simulink model "elevator"  (R2020a)
(part 3 of 38)

      mask DialogControl PLCBlockTitle Prompt: Examine If Closed (XIC)
  XIC3 : Subsystem  Priority=113  TreatAsAtomicUnit=on  mask{PLCOperandTag=F1PB, PLCBlockType=XIC, PLCPOUType=Contact, PLCOperandExpression=xxx_PLC_VAR_F1PB}
      mask prompts: PLCOperandTag "Operand Tag:"
      mask init:
      | slplc.callbacks.initInstruction(gcb);
      settings: AttributesFormatString=%<PLCOperandTag>
      mask Help: web([docroot '/plccoder/ref/xic' '.html']);
      mask DialogControl PLCBlockTitle Prompt: Examine If Closed (XIC)
  XIC30 : Subsystem  Priority=176  TreatAsAtomicUnit=on  mask{PLCOperandTag=F1PBHold, PLCBlockType=XIC, PLCPOUType=Contact, PLCOperandExpression=xxx_PLC_VAR_F1PBHold}
      mask prompts: PLCOperandTag "Operand Tag:"
      mask init:
      | slplc.callbacks.initInstruction(gcb);
      settings: AttributesFormatString=%<PLCOperandTag>
      mask Help: web([docroot '/plccoder/ref/xic' '.html']);
      mask DialogControl PLCBlockTitle Prompt: Examine If Closed (XIC)
  XIC31 : Subsystem  Priority=196  TreatAsAtomicUnit=on  mask{PLCOperandTag=StartHold, PLCBlockType=XIC, PLCPOUType=Contact, PLCOperandExpression=xxx_PLC_VAR_StartHold}
      mask prompts: PLCOperandTag "Operand Tag:"
      mask init:
      | slplc.callbacks.initInstruction(gcb);
      settings: AttributesFormatString=%<PLCOperandTag>
      mask Help: web([docroot '/plccoder/ref/xic' '.html']);
      mask DialogControl PLCBlockTitle Prompt: Examine If Closed (XIC)
  XIC32 : Subsystem  Priority=198  TreatAsAtomicUnit=on  mask{PLCOperandTag=LSTDIRUP, PLCBlockType=XIC, PLCPOUType=Contact, PLCOperandExpression=xxx_PLC_VAR_LSTDIRUP}
      mask prompts: PLCOperandTag "Operand Tag:"
      mask init:
      | slplc.callbacks.initInstruction(gcb);
      settings: AttributesFormatString=%<PLCOperandTag>
      mask Help: web([docroot '/plccoder/ref/xic' '.html']);
      mask DialogControl PLCBlockTitle Prompt: Examine If Closed (XIC)
  XIC33 : Subsystem  Priority=197  TreatAsAtomicUnit=on  mask{PLCOperandTag=GOINGUP, PLCBlockType=XIC, PLCPOUType=Contact, PLCOperandExpression=xxx_PLC_VAR_GOINGUP}
      mask prompts: PLCOperandTag "Operand Tag:"
      mask init:
      | slplc.callbacks.initInstruction(gcb);
      settings: AttributesFormatString=%<PLCOperandTag>
      mask Help: web([docroot '/plccoder/ref/xic' '.html']);
      mask DialogControl PLCBlockTitle Prompt: Examine If Closed (XIC)
  XIC34 : Subsystem  Priority=234  TreatAsAtomicUnit=on  mask{PLCOperandTag=MTRON, PLCBlockType=XIC, PLCPOUType=Contact, PLCOperandExpression=xxx_PLC_VAR_MTRON}
      mask prompts: PLCOperandTag "Operand Tag:"
      mask init:
      | slplc.callbacks.initInstruction(gcb);
      settings: AttributesFormatString=%<PLCOperandTag>
      mask Help: web([docroot '/plccoder/ref/xic' '.html']);
      mask DialogControl PLCBlockTitle Prompt: Examine If Closed (XIC)
  XIC35 : Subsystem  Priority=221  TreatAsAtomicUnit=on  mask{PLCOperandTag=F2PBHold, PLCBlockType=XIC, PLCPOUType=Contact, PLCOperandExpression=xxx_PLC_VAR_F2PBHold}
      mask prompts: PLCOperandTag "Operand Tag:"
      mask init:
      | slplc.callbacks.initInstruction(gcb);
      settings: AttributesFormatString=%<PLCOperandTag>
      mask Help: web([docroot '/plccoder/ref/xic' '.html']);
      mask DialogControl PLCBlockTitle Prompt: Examine If Closed (XIC)
  XIC36 : Subsystem  Priority=216  TreatAsAtomicUnit=on  mask{PLCOperandTag=F3DownBHold, PLCBlockType=XIC, PLCPOUType=Contact, PLCOperandExpression=xxx_PLC_VAR_F3DownBHold}
      mask prompts: PLCOperandTag "Operand Tag:"
      mask init:
      | slplc.callbacks.initInstruction(gcb);
      settings: AttributesFormatString=%<PLCOperandTag>
      mask Help: web([docroot '/plccoder/ref/xic' '.html']);
      mask DialogControl PLCBlockTitle Prompt: Examine If Closed (XIC)
  XIC37 : Subsystem  Priority=211  TreatAsAtomicUnit=on  mask{PLCOperandTag=F2PBHold, PLCBlockType=XIC, PLCPOUType=Contact, PLCOperandExpression=xxx_PLC_VAR_F2PBHold}
      mask prompts: PLCOperandTag "Operand Tag:"
      mask init:
      | slplc.callbacks.initInstruction(gcb);
      settings: AttributesFormatString=%<PLCOperandTag>
      mask Help: web([docroot '/plccoder/ref/xic' '.html']);
      mask DialogControl PLCBlockTitle Prompt: Examine If Closed (XIC)
  XIC38 : Subsystem  Priority=248  TreatAsAtomicUnit=on  mask{PLCOperandTag=MTRON, PLCBlockType=XIC, PLCPOUType=Contact, PLCOperandExpression=xxx_PLC_VAR_MTRON}
      mask prompts: PLCOperandTag "Operand Tag:"
      mask init:
      | slplc.callbacks.initInstruction(gcb);
      settings: AttributesFormatString=%<PLCOperandTag>
      mask Help: web([docroot '/plccoder/ref/xic' '.html']);
      mask DialogControl PLCBlockTitle Prompt: Examine If Closed (XIC)
  XIC39 : Subsystem  Priority=249  TreatAsAtomicUnit=on  mask{PLCOperandTag=RMPUPTRG, PLCBlockType=XIC, PLCPOUType=Contact, PLCOperandExpression=xxx_PLC_VAR_RMPUPTRG}
      mask prompts: PLCOperandTag "Operand Tag:"
      mask init:
      | slplc.callbacks.initInstruction(gcb);
      settings: AttributesFormatString=%<PLCOperandTag>
      mask Help: web([docroot '/plccoder/ref/xic' '.html']);
      mask DialogControl PLCBlockTitle Prompt: Examine If Closed (XIC)
  XIC4 : Subsystem  Priority=114  TreatAsAtomicUnit=on  mask{PLCOperandTag=F1PBHold, PLCBlockType=XIC, PLCPOUType=Contact, PLCOperandExpression=xxx_PLC_VAR_F1PBHold}
      mask prompts: PLCOperandTag "Operand Tag:"
      mask init:
      | slplc.callbacks.initInstruction(gcb);
      settings: AttributesFormatString=%<PLCOperandTag>
      mask Help: web([docroot '/plccoder/ref/xic' '.html']);
      mask DialogControl PLCBlockTitle Prompt: Examine If Closed (XIC)
  XIC40 : Subsystem  Priority=250  TreatAsAtomicUnit=on  mask{PLCOperandTag=RMPUP, PLCBlockType=XIC, PLCPOUType=Contact, PLCOperandExpression=xxx_PLC_VAR_RMPUP}
      mask prompts: PLCOperandTag "Operand Tag:"
      mask init:
      | slplc.callbacks.initInstruction(gcb);
      settings: AttributesFormatString=%<PLCOperandTag>
      mask Help: web([docroot '/plccoder/ref/xic' '.html']);
      mask DialogControl PLCBlockTitle Prompt: Examine If Closed (XIC)
  XIC41 : Subsystem  Priority=242  TreatAsAtomicUnit=on  mask{PLCOperandTag=SENCHK, PLCBlockType=XIC, PLCPOUType=Contact, PLCOperandExpression=xxx_PLC_VAR_SENCHK}
      mask prompts: PLCOperandTag "Operand Tag:"
      mask init:
      | slplc.callbacks.initInstruction(gcb);
      settings: AttributesFormatString=%<PLCOperandTag>
      mask Help: web([docroot '/plccoder/ref/xic' '.html']);
      mask DialogControl PLCBlockTitle Prompt: Examine If Closed (XIC)
  XIC42 : Subsystem  Priority=233  TreatAsAtomicUnit=on  mask{PLCOperandTag=StartHold, PLCBlockType=XIC, PLCPOUType=Contact, PLCOperandExpression=xxx_PLC_VAR_StartHold}
      mask prompts: PLCOperandTag "Operand Tag:"
      mask init:
      | slplc.callbacks.initInstruction(gcb);
      settings: AttributesFormatString=%<PLCOperandTag>
      mask Help: web([docroot '/plccoder/ref/xic' '.html']);
      mask DialogControl PLCBlockTitle Prompt: Examine If Closed (XIC)
  XIC43 : Subsystem  Priority=65  TreatAsAtomicUnit=on  mask{PLCOperandTag=TempS3LUp, PLCBlockType=XIC, PLCPOUType=Contact, PLCOperandExpression=xxx_PLC_VAR_TempS3LUp}
      mask prompts: PLCOperandTag "Operand Tag:"
      mask init:
      | slplc.callbacks.initInstruction(gcb);
      settings: AttributesFormatString=%<PLCOperandTag>
      mask Help: web([docroot '/plccoder/ref/xic' '.html']);
      mask DialogControl PLCBlockTitle Prompt: Examine If Closed (XIC)
  XIC44 : Subsystem  Priority=183  TreatAsAtomicUnit=on  mask{PLCOperandTag=MemoryGoUp, PLCBlockType=XIC, PLCPOUType=Contact, PLCOperandExpression=xxx_PLC_VAR_MemoryGoUp}
      mask prompts: PLCOperandTag "Operand Tag:"
      mask init:
      | slplc.callbacks.initInstruction(gcb);
      settings: AttributesFormatString=%<PLCOperandTag>
      mask Help: web([docroot '/plccoder/ref/xic' '.html']);
      mask DialogControl PLCBlockTitle Prompt: Examine If Closed (XIC)
  XIC45 : Subsystem  Priority=64  TreatAsAtomicUnit=on  mask{PLCOperandTag=StartHold, PLCBlockType=XIC, PLCPOUType=Contact, PLCOperandExpression=xxx_PLC_VAR_StartHold}
      mask prompts: PLCOperandTag "Operand Tag:"
      mask init:
      | slplc.callbacks.initInstruction(gcb);
      settings: AttributesFormatString=%<PLCOperandTag>
      mask Help: web([docroot '/plccoder/ref/xic' '.html']);
      mask DialogControl PLCBlockTitle Prompt: Examine If Closed (XIC)
  XIC46 : Subsystem  Priority=228  TreatAsAtomicUnit=on  mask{PLCOperandTag=S1H, PLCBlockType=XIC, PLCPOUType=Contact, PLCOperandExpression=xxx_PLC_VAR_S1H}
      mask prompts: PLCOperandTag "Operand Tag:"
      mask init:
      | slplc.callbacks.initInstruction(gcb);
      settings: AttributesFormatString=%<PLCOperandTag>
      mask Help: web([docroot '/plccoder/ref/xic' '.html']);
      mask DialogControl PLCBlockTitle Prompt: Examine If Closed (XIC)
  XIC47 : Subsystem  Priority=214  TreatAsAtomicUnit=on  mask{PLCOperandTag=S2L, PLCBlockType=XIC, PLCPOUType=Contact, PLCOperandExpression=xxx_PLC_VAR_S2L}
      mask prompts: PLCOperandTag "Operand Tag:"
      mask init:
      | slplc.callbacks.initInstruction(gcb);
      settings: AttributesFormatString=%<PLCOperandTag>
      mask Help: web([docroot '/plccoder/ref/xic' '.html']);
      mask DialogControl PLCBlockTitle Prompt: Examine If Closed (XIC)
  XIC48 : Subsystem  Priority=222  TreatAsAtomicUnit=on  mask{PLCOperandTag=F2UpDownBHold, PLCBlockType=XIC, PLCPOUType=Contact, PLCOperandExpression=xxx_PLC_VAR_F2UpDownBHold}
      mask prompts: PLCOperandTag "Operand Tag:"
      mask init:
      | slplc.callbacks.initInstruction(gcb);
      settings: AttributesFormatString=%<PLCOperandTag>
      mask Help: web([docroot '/plccoder/ref/xic' '.html']);
      mask DialogControl PLCBlockTitle Prompt: Examine If Closed (XIC)
  XIC49 : Subsystem  Priority=218  TreatAsAtomicUnit=on  mask{PLCOperandTag=S3L, PLCBlockType=XIC, PLCPOUType=Contact, PLCOperandExpression=xxx_PLC_VAR_S3L}
      mask prompts: PLCOperandTag "Operand Tag:"
      mask init:
      | slplc.callbacks.initInstruction(gcb);
      settings: AttributesFormatString=%<PLCOperandTag>
      mask Help: web([docroot '/plccoder/ref/xic' '.html']);
      mask DialogControl PLCBlockTitle Prompt: Examine If Closed (XIC)
  XIC5 : Subsystem  Priority=140  TreatAsAtomicUnit=on  mask{PLCOperandTag=StartHold, PLCBlockType=XIC, PLCPOUType=Contact, PLCOperandExpression=xxx_PLC_VAR_StartHold}
      mask prompts: PLCOperandTag "Operand Tag:"
      mask init:
      | slplc.callbacks.initInstruction(gcb);
      settings: AttributesFormatString=%<PLCOperandTag>
      mask Help: web([docroot '/plccoder/ref/xic' '.html']);
      mask DialogControl PLCBlockTitle Prompt: Examine If Closed (XIC)
  XIC50 : Subsystem  Priority=224  TreatAsAtomicUnit=on  mask{PLCOperandTag=S2H, PLCBlockType=XIC, PLCPOUType=Contact, PLCOperandExpression=xxx_PLC_VAR_S2H}
      mask prompts: PLCOperandTag "Operand Tag:"
      mask init:
      | slplc.callbacks.initInstruction(gcb);
      settings: AttributesFormatString=%<PLCOperandTag>
      mask Help: web([docroot '/plccoder/ref/xic' '.html']);
      mask DialogControl PLCBlockTitle Prompt: Examine If Closed (XIC)
  XIC51 : Subsystem  Priority=225  TreatAsAtomicUnit=on  mask{PLCOperandTag=F1PBHold, PLCBlockType=XIC, PLCPOUType=Contact, PLCOperandExpression=xxx_PLC_VAR_F1PBHold}
      mask prompts: PLCOperandTag "Operand Tag:"
      mask init:
      | slplc.callbacks.initInstruction(gcb);
      settings: AttributesFormatString=%<PLCOperandTag>
      mask Help: web([docroot '/plccoder/ref/xic' '.html']);
      mask DialogControl PLCBlockTitle Prompt: Examine If Closed (XIC)
  XIC52 : Subsystem  Priority=212  TreatAsAtomicUnit=on  mask{PLCOperandTag=F2UpDownBHold, PLCBlockType=XIC, PLCPOUType=Contact, PLCOperandExpression=xxx_PLC_VAR_F2UpDownBHold}
      mask prompts: PLCOperandTag "Operand Tag:"
      mask init:
      | slplc.callbacks.initInstruction(gcb);
      settings: AttributesFormatString=%<PLCOperandTag>
      mask Help: web([docroot '/plccoder/ref/xic' '.html']);
      mask DialogControl PLCBlockTitle Prompt: Examine If Closed (XIC)
  XIC53 : Subsystem  Priority=210  TreatAsAtomicUnit=on  mask{PLCOperandTag=GOINGUP, PLCBlockType=XIC, PLCPOUType=Contact, PLCOperandExpression=xxx_PLC_VAR_GOINGUP}
      mask prompts: PLCOperandTag "Operand Tag:"
      mask init:
      | slplc.callbacks.initInstruction(gcb);
      settings: AttributesFormatString=%<PLCOperandTag>
      mask Help: web([docroot '/plccoder/ref/xic' '.html']);
      mask DialogControl PLCBlockTitle Prompt: Examine If Closed (XIC)
  XIC54 : Subsystem  Priority=215  TreatAsAtomicUnit=on  mask{PLCOperandTag=F3PBHold, PLCBlockType=XIC, PLCPOUType=Contact, PLCOperandExpression=xxx_PLC_VAR_F3PBHold}
      mask prompts: PLCOperandTag "Operand Tag:"
      mask init:
      | slplc.callbacks.initInstruction(gcb);
      settings: AttributesFormatString=%<PLCOperandTag>
      mask Help: web([docroot '/plccoder/ref/xic' '.html']);
      mask DialogControl PLCBlockTitle Prompt: Examine If Closed (XIC)
  XIC55 : Subsystem  Priority=220  TreatAsAtomicUnit=on  mask{PLCOperandTag=GOINGDN, PLCBlockType=XIC, PLCPOUType=Contact, PLCOperandExpression=xxx_PLC_VAR_GOINGDN}
      mask prompts: PLCOperandTag "Operand Tag:"
      mask init:
      | slplc.callbacks.initInstruction(gcb);
      settings: AttributesFormatString=%<PLCOperandTag>
      mask Help: web([docroot '/plccoder/ref/xic' '.html']);
      mask DialogControl PLCBlockTitle Prompt: Examine If Closed (XIC)
  XIC56 : Subsystem  Priority=209  TreatAsAtomicUnit=on  mask{PLCOperandTag=StartHold, PLCBlockType=XIC, PLCPOUType=Contact, PLCOperandExpression=xxx_PLC_VAR_StartHold}
      mask prompts: PLCOperandTag "Operand Tag:"
      mask init:
      | slplc.callbacks.initInstruction(gcb);
      settings: AttributesFormatString=%<PLCOperandTag>
      mask Help: web([docroot '/plccoder/ref/xic' '.html']);
      mask DialogControl PLCBlockTitle Prompt: Examine If Closed (XIC)
  XIC57 : Subsystem  Priority=226  TreatAsAtomicUnit=on  mask{PLCOperandTag=F1UpBHold, PLCBlockType=XIC, PLCPOUType=Contact, PLCOperandExpression=xxx_PLC_VAR_F1UpBHold}
      mask prompts: PLCOperandTag "Operand Tag:"
      mask init:
      | slplc.callbacks.initInstruction(gcb);
      settings: AttributesFormatString=%<PLCOperandTag>
      mask Help: web([docroot '/plccoder/ref/xic' '.html']);
      mask DialogControl PLCBlockTitle Prompt: Examine If Closed (XIC)
  XIC58 : Subsystem  Priority=8  TreatAsAtomicUnit=on  mask{PLCOperandTag=StartHold, PLCBlockType=XIC, PLCPOUType=Contact, PLCOperandExpression=xxx_PLC_VAR_StartHold}
      mask prompts: PLCOperandTag "Operand Tag:"
      mask init:
      | slplc.callbacks.initInstruction(gcb);
      settings: AttributesFormatString=%<PLCOperandTag>
      mask Help: web([docroot '/plccoder/ref/xic' '.html']);
      mask DialogControl PLCBlockTitle Prompt: Examine If Closed (XIC)
  XIC59 : Subsystem  Priority=15  TreatAsAtomicUnit=on  mask{PLCOperandTag=StartHold, PLCBlockType=XIC, PLCPOUType=Contact, PLCOperandExpression=xxx_PLC_VAR_StartHold}
      mask prompts: PLCOperandTag "Operand Tag:"
      mask init:
      | slplc.callbacks.initInstruction(gcb);
      settings: AttributesFormatString=%<PLCOperandTag>
      mask Help: web([docroot '/plccoder/ref/xic' '.html']);
      mask DialogControl PLCBlockTitle Prompt: Examine If Closed (XIC)
  XIC6 : Subsystem  Priority=119  TreatAsAtomicUnit=on  mask{PLCOperandTag=StartHold, PLCBlockType=XIC, PLCPOUType=Contact, PLCOperandExpression=xxx_PLC_VAR_StartHold}
      mask prompts: PLCOperandTag "Operand Tag:"
      mask init:
      | slplc.callbacks.initInstruction(gcb);
      settings: AttributesFormatString=%<PLCOperandTag>
      mask Help: web([docroot '/plccoder/ref/xic' '.html']);
      mask DialogControl PLCBlockTitle Prompt: Examine If Closed (XIC)
  XIC60 : Subsystem  Priority=17  TreatAsAtomicUnit=on  mask{PLCOperandTag=S3L, PLCBlockType=XIC, PLCPOUType=Contact, PLCOperandExpression=xxx_PLC_VAR_S3L}
      mask prompts: PLCOperandTag "Operand Tag:"
      mask init:
      | slplc.callbacks.initInstruction(gcb);
      settings: AttributesFormatString=%<PLCOperandTag>
      mask Help: web([docroot '/plccoder/ref/xic' '.html']);
      mask DialogControl PLCBlockTitle Prompt: Examine If Closed (XIC)
  XIC61 : Subsystem  Priority=18  TreatAsAtomicUnit=on  mask{PLCOperandTag=TempS3LUp, PLCBlockType=XIC, PLCPOUType=Contact, PLCOperandExpression=xxx_PLC_VAR_TempS3LUp}
      mask prompts: PLCOperandTag "Operand Tag:"
      mask init:
      | slplc.callbacks.initInstruction(gcb);
      settings: AttributesFormatString=%<PLCOperandTag>
      mask Help: web([docroot '/plccoder/ref/xic' '.html']);
      mask DialogControl PLCBlockTitle Prompt: Examine If Closed (XIC)
  XIC62 : Subsystem  Priority=24  TreatAsAtomicUnit=on  mask{PLCOperandTag=S2H, PLCBlockType=XIC, PLCPOUType=Contact, PLCOperandExpression=xxx_PLC_VAR_S2H}
      mask prompts: PLCOperandTag "Operand Tag:"
      mask init:
      | slplc.callbacks.initInstruction(gcb);
      settings: AttributesFormatString=%<PLCOperandTag>
      mask Help: web([docroot '/plccoder/ref/xic' '.html']);
      mask DialogControl PLCBlockTitle Prompt: Examine If Closed (XIC)
  XIC63 : Subsystem  Priority=25  TreatAsAtomicUnit=on  mask{PLCOperandTag=TempS2HDown, PLCBlockType=XIC, PLCPOUType=Contact, PLCOperandExpression=xxx_PLC_VAR_TempS2HDown}
      mask prompts: PLCOperandTag "Operand Tag:"
      mask init:
      | slplc.callbacks.initInstruction(gcb);
      settings: AttributesFormatString=%<PLCOperandTag>
      mask Help: web([docroot '/plccoder/ref/xic' '.html']);
      mask DialogControl PLCBlockTitle Prompt: Examine If Closed (XIC)
  XIC64 : Subsystem  Priority=38  TreatAsAtomicUnit=on  mask{PLCOperandTag=S2L, PLCBlockType=XIC, PLCPOUType=Contact, PLCOperandExpression=xxx_PLC_VAR_S2L}
      mask prompts: PLCOperandTag "Operand Tag:"
      mask init:
      | slplc.callbacks.initInstruction(gcb);
      settings: AttributesFormatString=%<PLCOperandTag>
      mask Help: web([docroot '/plccoder/ref/xic' '.html']);
      mask DialogControl PLCBlockTitle Prompt: Examine If Closed (XIC)
  XIC65 : Subsystem  Priority=39  TreatAsAtomicUnit=on  mask{PLCOperandTag=TempS2LDown, PLCBlockType=XIC, PLCPOUType=Contact, PLCOperandExpression=xxx_PLC_VAR_TempS2LDown}
      mask prompts: PLCOperandTag "Operand Tag:"
      mask init:
      | slplc.callbacks.initInstruction(gcb);
      settings: AttributesFormatString=%<PLCOperandTag>
      mask Help: web([docroot '/plccoder/ref/xic' '.html']);
      mask DialogControl PLCBlockTitle Prompt: Examine If Closed (XIC)
  XIC66 : Subsystem  Priority=52  TreatAsAtomicUnit=on  mask{PLCOperandTag=S1H, PLCBlockType=XIC, PLCPOUType=Contact, PLCOperandExpression=xxx_PLC_VAR_S1H}
      mask prompts: PLCOperandTag "Operand Tag:"
      mask init:
      | slplc.callbacks.initInstruction(gcb);
      settings: AttributesFormatString=%<PLCOperandTag>
      mask Help: web([docroot '/plccoder/ref/xic' '.html']);
      mask DialogControl PLCBlockTitle Prompt: Examine If Closed (XIC)
  XIC67 : Subsystem  Priority=53  TreatAsAtomicUnit=on  mask{PLCOperandTag=TempS1HDown, PLCBlockType=XIC, PLCPOUType=Contact, PLCOperandExpression=xxx_PLC_VAR_TempS1HDown}
      mask prompts: PLCOperandTag "Operand Tag:"
      mask init:
      | slplc.callbacks.initInstruction(gcb);
      settings: AttributesFormatString=%<PLCOperandTag>
      mask Help: web([docroot '/plccoder/ref/xic' '.html']);
      mask DialogControl PLCBlockTitle Prompt: Examine If Closed (XIC)
  XIC68 : Subsystem  Priority=36  TreatAsAtomicUnit=on  mask{PLCOperandTag=StartHold, PLCBlockType=XIC, PLCPOUType=Contact, PLCOperandExpression=xxx_PLC_VAR_StartHold}
      mask prompts: PLCOperandTag "Operand Tag:"
      mask init:
      | slplc.callbacks.initInstruction(gcb);
      settings: AttributesFormatString=%<PLCOperandTag>
      mask Help: web([docroot '/plccoder/ref/xic' '.html']);
      mask DialogControl PLCBlockTitle Prompt: Examine If Closed (XIC)
  XIC69 : Subsystem  Priority=43  TreatAsAtomicUnit=on  mask{PLCOperandTag=StartHold, PLCBlockType=XIC, PLCPOUType=Contact, PLCOperandExpression=xxx_PLC_VAR_StartHold}
      mask prompts: PLCOperandTag "Operand Tag:"
      mask init:
      | slplc.callbacks.initInstruction(gcb);
      settings: AttributesFormatString=%<PLCOperandTag>
      mask Help: web([docroot '/plccoder/ref/xic' '.html']);
      mask DialogControl PLCBlockTitle Prompt: Examine If Closed (XIC)
  XIC7 : Subsystem  Priority=120  TreatAsAtomicUnit=on  mask{PLCOperandTag=F2PB, PLCBlockType=XIC, PLCPOUType=Contact, PLCOperandExpression=xxx_PLC_VAR_F2PB}
      mask prompts: PLCOperandTag "Operand Tag:"
      mask init:
      | slplc.callbacks.initInstruction(gcb);
      settings: AttributesFormatString=%<PLCOperandTag>
      mask Help: web([docroot '/plccoder/ref/xic' '.html']);
      mask DialogControl PLCBlockTitle Prompt: Examine If Closed (XIC)
  XIC70 : Subsystem  Priority=16  TreatAsAtomicUnit=on  mask{PLCOperandTag=TempS2HUp, PLCBlockType=XIC, PLCPOUType=Contact, PLCOperandExpression=xxx_PLC_VAR_TempS2HUp}
      mask prompts: PLCOperandTag "Operand Tag:"
      mask init:
      | slplc.callbacks.initInstruction(gcb);
      settings: AttributesFormatString=%<PLCOperandTag>
      mask Help: web([docroot '/plccoder/ref/xic' '.html']);
      mask DialogControl PLCBlockTitle Prompt: Examine If Closed (XIC)
  XIC71 : Subsystem  Priority=57  TreatAsAtomicUnit=on  mask{PLCOperandTag=StartHold, PLCBlockType=XIC, PLCPOUType=Contact, PLCOperandExpression=xxx_PLC_VAR_StartHold}
      mask prompts: PLCOperandTag "Operand Tag:"
      mask init:
      | slplc.callbacks.initInstruction(gcb);
      settings: AttributesFormatString=%<PLCOperandTag>
      mask Help: web([docroot '/plccoder/ref/xic' '.html']);
      mask DialogControl PLCBlockTitle Prompt: Examine If Closed (XIC)
  XIC72 : Subsystem  Priority=29  TreatAsAtomicUnit=on  mask{PLCOperandTag=StartHold, PLCBlockType=XIC, PLCPOUType=Contact, PLCOperandExpression=xxx_PLC_VAR_StartHold}
      mask prompts: PLCOperandTag "Operand Tag:"
      mask init:
      | slplc.callbacks.initInstruction(gcb);
      settings: AttributesFormatString=%<PLCOperandTag>
      mask Help: web([docroot '/plccoder/ref/xic' '.html']);
      mask DialogControl PLCBlockTitle Prompt: Examine If Closed (XIC)
  XIC73 : Subsystem  Priority=182  TreatAsAtomicUnit=on  mask{PLCOperandTag=StartHold, PLCBlockType=XIC, PLCPOUType=Contact, PLCOperandExpression=xxx_PLC_VAR_StartHold}
      mask prompts: PLCOperandTag "Operand Tag:"
      mask init:
      | slplc.callbacks.initInstruction(gcb);
      settings: AttributesFormatString=%<PLCOperandTag>
      mask Help: web([docroot '/plccoder/ref/xic' '.html']);
      mask DialogControl PLCBlockTitle Prompt: Examine If Closed (XIC)
  XIC74 : Subsystem  Priority=104  TreatAsAtomicUnit=on  mask{PLCOperandTag=StartHold, PLCBlockType=XIC, PLCPOUType=Contact, PLCOperandExpression=xxx_PLC_VAR_StartHold}
      mask prompts: PLCOperandTag "Operand Tag:"
      mask init:
      | slplc.callbacks.initInstruction(gcb);
      settings: AttributesFormatString=%<PLCOperandTag>
      mask Help: web([docroot '/plccoder/ref/xic' '.html']);
      mask DialogControl PLCBlockTitle Prompt: Examine If Closed (XIC)
  XIC75 : Subsystem  Priority=96  TreatAsAtomicUnit=on  mask{PLCOperandTag=StartHold, PLCBlockType=XIC, PLCPOUType=Contact, PLCOperandExpression=xxx_PLC_VAR_StartHold}
      mask prompts: PLCOperandTag "Operand Tag:"
      mask init:
      | slplc.callbacks.initInstruction(gcb);
      settings: AttributesFormatString=%<PLCOperandTag>
      mask Help: web([docroot '/plccoder/ref/xic' '.html']);
      mask DialogControl PLCBlockTitle Prompt: Examine If Closed (XIC)
  XIC76 : Subsystem  Priority=88  TreatAsAtomicUnit=on  mask{PLCOperandTag=StartHold, PLCBlockType=XIC, PLCPOUType=Contact, PLCOperandExpression=xxx_PLC_VAR_StartHold}
      mask prompts: PLCOperandTag "Operand Tag:"
      mask init:
      | slplc.callbacks.initInstruction(gcb);
      settings: AttributesFormatString=%<PLCOperandTag>
      mask Help: web([docroot '/plccoder/ref/xic' '.html']);
      mask DialogControl PLCBlockTitle Prompt: Examine If Closed (XIC)
  XIC77 : Subsystem  Priority=51  TreatAsAtomicUnit=on  mask{PLCOperandTag=TempS2LDown, PLCBlockType=XIC, PLCPOUType=Contact, PLCOperandExpression=xxx_PLC_VAR_TempS2LDown}
      mask prompts: PLCOperandTag "Operand Tag:"
      mask init:
      | slplc.callbacks.initInstruction(gcb);
      settings: AttributesFormatString=%<PLCOperandTag>
      mask Help: web([docroot '/plccoder/ref/xic' '.html']);
      mask DialogControl PLCBlockTitle Prompt: Examine If Closed (XIC)
  XIC78 : Subsystem  Priority=50  TreatAsAtomicUnit=on  mask{PLCOperandTag=StartHold, PLCBlockType=XIC, PLCPOUType=Contact, PLCOperandExpression=xxx_PLC_VAR_StartHold}
      mask prompts: PLCOperandTag "Operand Tag:"
      mask init:
      | slplc.callbacks.initInstruction(gcb);
      settings: AttributesFormatString=%<PLCOperandTag>
      mask Help: web([docroot '/plccoder/ref/xic' '.html']);
      mask DialogControl PLCBlockTitle Prompt: Examine If Closed (XIC)
  XIC79 : Subsystem  Priority=82  TreatAsAtomicUnit=on  mask{PLCOperandTag=TempS1HDown, PLCBlockType=XIC, PLCPOUType=Contact, PLCOperandExpression=xxx_PLC_VAR_TempS1HDown}
      mask prompts: PLCOperandTag "Operand Tag:"
      mask init:
      | slplc.callbacks.initInstruction(gcb);
      settings: AttributesFormatString=%<PLCOperandTag>
      mask Help: web([docroot '/plccoder/ref/xic' '.html']);
      mask DialogControl PLCBlockTitle Prompt: Examine If Closed (XIC)
  XIC8 : Subsystem  Priority=121  TreatAsAtomicUnit=on  mask{PLCOperandTag=F2PBHold, PLCBlockType=XIC, PLCPOUType=Contact, PLCOperandExpression=xxx_PLC_VAR_F2PBHold}
      mask prompts: PLCOperandTag "Operand Tag:"
      mask init:
      | slplc.callbacks.initInstruction(gcb);
      settings: AttributesFormatString=%<PLCOperandTag>
      mask Help: web([docroot '/plccoder/ref/xic' '.html']);
      mask DialogControl PLCBlockTitle Prompt: Examine If Closed (XIC)
  XIC80 : Subsystem  Priority=81  TreatAsAtomicUnit=on  mask{PLCOperandTag=StartHold, PLCBlockType=XIC, PLCPOUType=Contact, PLCOperandExpression=xxx_PLC_VAR_StartHold}
      mask prompts: PLCOperandTag "Operand Tag:"
      mask init:
      | slplc.callbacks.initInstruction(gcb);
      settings: AttributesFormatString=%<PLCOperandTag>
      mask Help: web([docroot '/plccoder/ref/xic' '.html']);
      mask DialogControl PLCBlockTitle Prompt: Examine If Closed (XIC)
  XIC81 : Subsystem  Priority=22  TreatAsAtomicUnit=on  mask{PLCOperandTag=StartHold, PLCBlockType=XIC, PLCPOUType=Contact, PLCOperandExpression=xxx_PLC_VAR_StartHold}
      mask prompts: PLCOperandTag "Operand Tag:"
      mask init:
      | slplc.callbacks.initInstruction(gcb);
      settings: AttributesFormatString=%<PLCOperandTag>
      mask Help: web([docroot '/plccoder/ref/xic' '.html']);
      mask DialogControl PLCBlockTitle Prompt: Examine If Closed (XIC)
  XIC82 : Subsystem  Priority=23  TreatAsAtomicUnit=on  mask{PLCOperandTag=TempS3LDown, PLCBlockType=XIC, PLCPOUType=Contact, PLCOperandExpression=xxx_PLC_VAR_TempS3LDown}
      mask prompts: PLCOperandTag "Operand Tag:"
      mask init:
      | slplc.callbacks.initInstruction(gcb);
      settings: AttributesFormatString=%<PLCOperandTag>
      mask Help: web([docroot '/plccoder/ref/xic' '.html']);
      mask DialogControl PLCBlockTitle Prompt: Examine If Closed (XIC)
  XIC83 : Subsystem  Priority=71  TreatAsAtomicUnit=on  mask{PLCOperandTag=StartHold, PLCBlockType=XIC, PLCPOUType=Contact, PLCOperandExpression=xxx_PLC_VAR_StartHold}
      mask prompts: PLCOperandTag "Operand Tag:"
      mask init:
      | slplc.callbacks.initInstruction(gcb);
      settings: AttributesFormatString=%<PLCOperandTag>
      mask Help: web([docroot '/plccoder/ref/xic' '.html']);
      mask DialogControl PLCBlockTitle Prompt: Examine If Closed (XIC)
  XIC84 : Subsystem  Priority=74  TreatAsAtomicUnit=on  mask{PLCOperandTag=TempS2LUp, PLCBlockType=XIC, PLCPOUType=Contact, PLCOperandExpression=xxx_PLC_VAR_TempS2LUp}
      mask prompts: PLCOperandTag "Operand Tag:"
      mask init:
      | slplc.callbacks.initInstruction(gcb);
      settings: AttributesFormatString=%<PLCOperandTag>
      mask Help: web([docroot '/plccoder/ref/xic' '.html']);
      mask DialogControl PLCBlockTitle Prompt: Examine If Closed (XIC)
  XIC85 : Subsystem  Priority=59  TreatAsAtomicUnit=on  mask{PLCOperandTag=S1H, PLCBlockType=XIC, PLCPOUType=Contact, PLCOperandExpression=xxx_PLC_VAR_S1H}
      mask prompts: PLCOperandTag "Operand Tag:"
      mask init:
      | slplc.callbacks.initInstruction(gcb);
      settings: AttributesFormatString=%<PLCOperandTag>
      mask Help: web([docroot '/plccoder/ref/xic' '.html']);
      mask DialogControl PLCBlockTitle Prompt: Examine If Closed (XIC)
  XIC86 : Subsystem  Priority=44  TreatAsAtomicUnit=on  mask{PLCOperandTag=TempS1HUp, PLCBlockType=XIC, PLCPOUType=Contact, PLCOperandExpression=xxx_PLC_VAR_TempS1HUp}
      mask prompts: PLCOperandTag "Operand Tag:"
      mask init:
      | slplc.callbacks.initInstruction(gcb);
      settings: AttributesFormatString=%<PLCOperandTag>
      mask Help: web([docroot '/plccoder/ref/xic' '.html']);
      mask DialogControl PLCBlockTitle Prompt: Examine If Closed (XIC)
  XIC87 : Subsystem  Priority=72  TreatAsAtomicUnit=on  mask{PLCOperandTag=TempS2HDown, PLCBlockType=XIC, PLCPOUType=Contact, PLCOperandExpression=xxx_PLC_VAR_TempS2HDown}
      mask prompts: PLCOperandTag "Operand Tag:"
      mask init:
      | slplc.callbacks.initInstruction(gcb);
      settings: AttributesFormatString=%<PLCOperandTag>
      mask Help: web([docroot '/plccoder/ref/xic' '.html']);
      mask DialogControl PLCBlockTitle Prompt: Examine If Closed (XIC)
  XIC88 : Subsystem  Priority=60  TreatAsAtomicUnit=on  mask{PLCOperandTag=TempS1HUp, PLCBlockType=XIC, PLCPOUType=Contact, PLCOperandExpression=xxx_PLC_VAR_TempS1HUp}
      mask prompts: PLCOperandTag "Operand Tag:"
      mask init:
      | slplc.callbacks.initInstruction(gcb);
      settings: AttributesFormatString=%<PLCOperandTag>
      mask Help: web([docroot '/plccoder/ref/xic' '.html']);
      mask DialogControl PLCBlockTitle Prompt: Examine If Closed (XIC)
  XIC89 : Subsystem  Priority=184  TreatAsAtomicUnit=on  mask{PLCOperandTag=LSTDIRUP, PLCBlockType=XIC, PLCPOUType=Contact, PLCOperandExpression=xxx_PLC_VAR_LSTDIRUP}
      mask prompts: PLCOperandTag "Operand Tag:"
      mask init:
      | slplc.callbacks.initInstruction(gcb);
      settings: AttributesFormatString=%<PLCOperandTag>
      mask Help: web([docroot '/plccoder/ref/xic' '.html']);
      mask DialogControl PLCBlockTitle Prompt: Examine If Closed (XIC)
  XIC9 : Subsystem  Priority=141  TreatAsAtomicUnit=on  mask{PLCOperandTag=F2UpB, PLCBlockType=XIC, PLCPOUType=Contact, PLCOperandExpression=xxx_PLC_VAR_F2UpB}
      mask prompts: PLCOperandTag "Operand Tag:"
      mask init:
      | slplc.callbacks.initInstruction(gcb);
      settings: AttributesFormatString=%<PLCOperandTag>
      mask Help: web([docroot '/plccoder/ref/xic' '.html']);
      mask DialogControl PLCBlockTitle Prompt: Examine If Closed (XIC)
  XIC90 : Subsystem  Priority=45  TreatAsAtomicUnit=on  mask{PLCOperandTag=S2L, PLCBlockType=XIC, PLCPOUType=Contact, PLCOperandExpression=xxx_PLC_VAR_S2L}
      mask prompts: PLCOperandTag "Operand Tag:"
      mask init:
      | slplc.callbacks.initInstruction(gcb);
      settings: AttributesFormatString=%<PLCOperandTag>
      mask Help: web([docroot '/plccoder/ref/xic' '.html']);
      mask DialogControl PLCBlockTitle Prompt: Examine If Closed (XIC)
  XIC91 : Subsystem  Priority=46  TreatAsAtomicUnit=on  mask{PLCOperandTag=TempS2LUp, PLCBlockType=XIC, PLCPOUType=Contact, PLCOperandExpression=xxx_PLC_VAR_TempS2LUp}
      mask prompts: PLCOperandTag "Operand Tag:"
      mask init:
      | slplc.callbacks.initInstruction(gcb);
      settings: AttributesFormatString=%<PLCOperandTag>
      mask Help: web([docroot '/plccoder/ref/xic' '.html']);
      mask DialogControl PLCBlockTitle Prompt: Examine If Closed (XIC)
  XIC92 : Subsystem  Priority=204  TreatAsAtomicUnit=on  mask{PLCOperandTag=GOINGUP, PLCBlockType=XIC, PLCPOUType=Contact, PLCOperandExpression=xxx_PLC_VAR_GOINGUP}
      mask prompts: PLCOperandTag "Operand Tag:"
      mask init:
      | slplc.callbacks.initInstruction(gcb);
      settings: AttributesFormatString=%<PLCOperandTag>
      mask Help: web([docroot '/plccoder/ref/xic' '.html']);
      mask DialogControl PLCBlockTitle Prompt: Examine If Closed (XIC)
  XIC93 : Subsystem  Priority=31  TreatAsAtomicUnit=on  mask{PLCOperandTag=S2H, PLCBlockType=XIC, PLCPOUType=Contact, PLCOperandExpression=xxx_PLC_VAR_S2H}
      mask prompts: PLCOperandTag "Operand Tag:"
      mask init:
      | slplc.callbacks.initInstruction(gcb);
      settings: AttributesFormatString=%<PLCOperandTag>
      mask Help: web([docroot '/plccoder/ref/xic' '.html']);
      mask DialogControl PLCBlockTitle Prompt: Examine If Closed (XIC)
  XIC94 : Subsystem  Priority=32  TreatAsAtomicUnit=on  mask{PLCOperandTag=TempS2HUp, PLCBlockType=XIC, PLCPOUType=Contact, PLCOperandExpression=xxx_PLC_VAR_TempS2HUp}
      mask prompts: PLCOperandTag "Operand Tag:"
      mask init:
      | slplc.callbacks.initInstruction(gcb);
      settings: AttributesFormatString=%<PLCOperandTag>
      mask Help: web([docroot '/plccoder/ref/xic' '.html']);
      mask DialogControl PLCBlockTitle Prompt: Examine If Closed (XIC)
  XIC95 : Subsystem  Priority=10  TreatAsAtomicUnit=on  mask{PLCOperandTag=S3L, PLCBlockType=XIC, PLCPOUType=Contact, PLCOperandExpression=xxx_PLC_VAR_S3L}
      mask prompts: PLCOperandTag "Operand Tag:"
      mask init:
      | slplc.callbacks.initInstruction(gcb);
      settings: AttributesFormatString=%<PLCOperandTag>
      mask Help: web([docroot '/plccoder/ref/xic' '.html']);
      mask DialogControl PLCBlockTitle Prompt: Examine If Closed (XIC)
  XIC96 : Subsystem  Priority=11  TreatAsAtomicUnit=on  mask{PLCOperandTag=TempS3LDown, PLCBlockType=XIC, PLCPOUType=Contact, PLCOperandExpression=xxx_PLC_VAR_TempS3LDown}
      mask prompts: PLCOperandTag "Operand Tag:"
      mask init:
      | slplc.callbacks.initInstruction(gcb);
      settings: AttributesFormatString=%<PLCOperandTag>
      mask Help: web([docroot '/plccoder/ref/xic' '.html']);
      mask DialogControl PLCBlockTitle Prompt: Examine If Closed (XIC)
  XIC97 : Subsystem  Priority=190  TreatAsAtomicUnit=on  mask{PLCOperandTag=MemoryGoDown, PLCBlockType=XIC, PLCPOUType=Contact, PLCOperandExpression=xxx_PLC_VAR_MemoryGoDown}
      mask prompts: PLCOperandTag "Operand Tag:"
      mask init:
      | slplc.callbacks.initInstruction(gcb);
      settings: AttributesFormatString=%<PLCOperandTag>
      mask Help: web([docroot '/plccoder/ref/xic' '.html']);
      mask DialogControl PLCBlockTitle Prompt: Examine If Closed (XIC)
  XIC98 : Subsystem  Priority=189  TreatAsAtomicUnit=on  mask{PLCOperandTag=StartHold, PLCBlockType=XIC, PLCPOUType=Contact, PLCOperandExpression=xxx_PLC_VAR_StartHold}
      mask prompts: PLCOperandTag "Operand Tag:"
      mask init:
      | slplc.callbacks.initInstruction(gcb);
      settings: AttributesFormatString=%<PLCOperandTag>
      mask Help: web([docroot '/plccoder/ref/xic' '.html']);
      mask DialogControl PLCBlockTitle Prompt: Examine If Closed (XIC)
  XIC99 : Subsystem  Priority=203  TreatAsAtomicUnit=on  mask{PLCOperandTag=StartHold, PLCBlockType=XIC, PLCPOUType=Contact, PLCOperandExpression=xxx_PLC_VAR_StartHold}
      mask prompts: PLCOperandTag "Operand Tag:"
      mask init:
      | slplc.callbacks.initInstruction(gcb);
      settings: AttributesFormatString=%<PLCOperandTag>
      mask Help: web([docroot '/plccoder/ref/xic' '.html']);
      mask DialogControl PLCBlockTitle Prompt: Examine If Closed (XIC)
  XIO : Subsystem  Priority=5  TreatAsAtomicUnit=on  mask{PLCOperandExpression=xxx_PLC_VAR_Stop, PLCOperandTag=Stop, PLCBlockType=XIO, PLCPOUType=Contact}
      mask prompts: PLCOperandTag "Operand Tag:"
      mask init:
      | slplc.callbacks.initInstruction(gcb);
      settings: AttributesFormatString=%<PLCOperandTag>
      mask Help: web([docroot '/plccoder/ref/xio' '.html']);
      mask DialogControl PLCBlockTitle Prompt: Examine If Open (XIO)
  XIO1 : Subsystem  Priority=116  TreatAsAtomicUnit=on  mask{PLCOperandExpression=xxx_PLC_VAR_AtFloor1, PLCOperandTag=AtFloor1, PLCBlockType=XIO, PLCPOUType=Contact}
      mask prompts: PLCOperandTag "Operand Tag:"
      mask init:
      | slplc.callbacks.initInstruction(gcb);
      settings: AttributesFormatString=%<PLCOperandTag>
      mask Help: web([docroot '/plccoder/ref/xio' '.html']);
      mask DialogControl PLCBlockTitle Prompt: Examine If Open (XIO)
  XIO10 : Subsystem  Priority=173  TreatAsAtomicUnit=on  mask{PLCOperandExpression=xxx_PLC_VAR_AtFloor1, PLCOperandTag=AtFloor1, PLCBlockType=XIO, PLCPOUType=Contact}
      mask prompts: PLCOperandTag "Operand Tag:"
      mask init:
      | slplc.callbacks.initInstruction(gcb);
      settings: AttributesFormatString=%<PLCOperandTag>
      mask Help: web([docroot '/plccoder/ref/xio' '.html']);
      mask DialogControl PLCBlockTitle Prompt: Examine If Open (XIO)
  XIO11 : Subsystem  Priority=174  TreatAsAtomicUnit=on  mask{PLCOperandExpression=xxx_PLC_VAR_AtFloor2, PLCOperandTag=AtFloor2, PLCBlockType=XIO, PLCPOUType=Contact}
      mask prompts: PLCOperandTag "Operand Tag:"
      mask init:
      | slplc.callbacks.initInstruction(gcb);
      settings: AttributesFormatString=%<PLCOperandTag>
      mask Help: web([docroot '/plccoder/ref/xio' '.html']);
      mask DialogControl PLCBlockTitle Prompt: Examine If Open (XIO)
  XIO12 : Subsystem  Priority=178  TreatAsAtomicUnit=on  mask{PLCOperandExpression=xxx_PLC_VAR_AtFloor1, PLCOperandTag=AtFloor1, PLCBlockType=XIO, PLCPOUType=Contact}
      mask prompts: PLCOperandTag "Operand Tag:"
      mask init:
      | slplc.callbacks.initInstruction(gcb);
      settings: AttributesFormatString=%<PLCOperandTag>
      mask Help: web([docroot '/plccoder/ref/xio' '.html']);
      mask DialogControl PLCBlockTitle Prompt: Examine If Open (XIO)
  XIO13 : Subsystem  Priority=73  TreatAsAtomicUnit=on  mask{PLCOperandExpression=xxx_PLC_VAR_S2H, PLCOperandTag=S2H, PLCBlockType=XIO, PLCPOUType=Contact}
      mask prompts: PLCOperandTag "Operand Tag:"
      mask init:
      | slplc.callbacks.initInstruction(gcb);
      settings: AttributesFormatString=%<PLCOperandTag>
      mask Help: web([docroot '/plccoder/ref/xio' '.html']);
      mask DialogControl PLCBlockTitle Prompt: Examine If Open (XIO)
  XIO14 : Subsystem  Priority=75  TreatAsAtomicUnit=on  mask{PLCOperandExpression=xxx_PLC_VAR_S2L, PLCOperandTag=S2L, PLCBlockType=XIO, PLCPOUType=Contact}
      mask prompts: PLCOperandTag "Operand Tag:"
      mask init:
      | slplc.callbacks.initInstruction(gcb);
      settings: AttributesFormatString=%<PLCOperandTag>
      mask Help: web([docroot '/plccoder/ref/xio' '.html']);
      mask DialogControl PLCBlockTitle Prompt: Examine If Open (XIO)
  XIO15 : Subsystem  Priority=83  TreatAsAtomicUnit=on  mask{PLCOperandExpression=xxx_PLC_VAR_S1H, PLCOperandTag=S1H, PLCBlockType=XIO, PLCPOUType=Contact}
      mask prompts: PLCOperandTag "Operand Tag:"
      mask init:
      | slplc.callbacks.initInstruction(gcb);
      settings: AttributesFormatString=%<PLCOperandTag>
      mask Help: web([docroot '/plccoder/ref/xio' '.html']);
      mask DialogControl PLCBlockTitle Prompt: Examine If Open (XIO)
  XIO16 : Subsystem  Priority=66  TreatAsAtomicUnit=on  mask{PLCOperandExpression=xxx_PLC_VAR_S3L, PLCOperandTag=S3L, PLCBlockType=XIO, PLCPOUType=Contact}
      mask prompts: PLCOperandTag "Operand Tag:"
      mask init:
      | slplc.callbacks.initInstruction(gcb);
      settings: AttributesFormatString=%<PLCOperandTag>
      mask Help: web([docroot '/plccoder/ref/xio' '.html']);
      mask DialogControl PLCBlockTitle Prompt: Examine If Open (XIO)
  XIO17 : Subsystem  Priority=185  TreatAsAtomicUnit=on  mask{PLCOperandExpression=xxx_PLC_VAR_MemoryGoDown, PLCOperandTag=MemoryGoDown, PLCBlockType=XIO, PLCPOUType=Contact}
      mask prompts: PLCOperandTag "Operand Tag:"
      mask init:
      | slplc.callbacks.initInstruction(gcb);
      settings: AttributesFormatString=%<PLCOperandTag>
      mask Help: web([docroot '/plccoder/ref/xio' '.html']);
      mask DialogControl PLCBlockTitle Prompt: Examine If Open (XIO)
  XIO18 : Subsystem  Priority=106  TreatAsAtomicUnit=on  mask{PLCOperandExpression=xxx_PLC_VAR_AtFloor3, PLCOperandTag=AtFloor3, PLCBlockType=XIO, PLCPOUType=Contact}
      mask prompts: PLCOperandTag "Operand Tag:"
      mask init:
      | slplc.callbacks.initInstruction(gcb);
      settings: AttributesFormatString=%<PLCOperandTag>
      mask Help: web([docroot '/plccoder/ref/xio' '.html']);
      mask DialogControl PLCBlockTitle Prompt: Examine If Open (XIO)
  XIO19 : Subsystem  Priority=105  TreatAsAtomicUnit=on  mask{PLCOperandExpression=xxx_PLC_VAR_AtFloor2, PLCOperandTag=AtFloor2, PLCBlockType=XIO, PLCPOUType=Contact}
      mask prompts: PLCOperandTag "Operand Tag:"
      mask init:
      | slplc.callbacks.initInstruction(gcb);
      settings: AttributesFormatString=%<PLCOperandTag>
      mask Help: web([docroot '/plccoder/ref/xio' '.html']);
      mask DialogControl PLCBlockTitle Prompt: Examine If Open (XIO)
  XIO2 : Subsystem  Priority=123  TreatAsAtomicUnit=on  mask{PLCOperandExpression=xxx_PLC_VAR_AtFloor2, PLCOperandTag=AtFloor2, PLCBlockType=XIO, PLCPOUType=Contact}
      mask prompts: PLCOperandTag "Operand Tag:"
      mask init:
      | slplc.callbacks.initInstruction(gcb);
      settings: AttributesFormatString=%<PLCOperandTag>
      mask Help: web([docroot '/plccoder/ref/xio' '.html']);
      mask DialogControl PLCBlockTitle Prompt: Examine If Open (XIO)
  XIO20 : Subsystem  Priority=97  TreatAsAtomicUnit=on  mask{PLCOperandExpression=xxx_PLC_VAR_AtFloor1, PLCOperandTag=AtFloor1, PLCBlockType=XIO, PLCPOUType=Contact}
      mask prompts: PLCOperandTag "Operand Tag:"
      mask init:
      | slplc.callbacks.initInstruction(gcb);
      settings: AttributesFormatString=%<PLCOperandTag>
      mask Help: web([docroot '/plccoder/ref/xio' '.html']);
      mask DialogControl PLCBlockTitle Prompt: Examine If Open (XIO)
  XIO21 : Subsystem  Priority=98  TreatAsAtomicUnit=on  mask{PLCOperandExpression=xxx_PLC_VAR_AtFloor3, PLCOperandTag=AtFloor3, PLCBlockType=XIO, PLCPOUType=Contact}
      mask prompts: PLCOperandTag "Operand Tag:"
      mask init:
      | slplc.callbacks.initInstruction(gcb);
      settings: AttributesFormatString=%<PLCOperandTag>
      mask Help: web([docroot '/plccoder/ref/xio' '.html']);
      mask DialogControl PLCBlockTitle Prompt: Examine If Open (XIO)
  XIO22 : Subsystem  Priority=89  TreatAsAtomicUnit=on  mask{PLCOperandExpression=xxx_PLC_VAR_AtFloor1, PLCOperandTag=AtFloor1, PLCBlockType=XIO, PLCPOUType=Contact}
      mask prompts: PLCOperandTag "Operand Tag:"
      mask init:
      | slplc.callbacks.initInstruction(gcb);
      settings: AttributesFormatString=%<PLCOperandTag>
      mask Help: web([docroot '/plccoder/ref/xio' '.html']);
      mask DialogControl PLCBlockTitle Prompt: Examine If Open (XIO)
  XIO23 : Subsystem  Priority=37  TreatAsAtomicUnit=on  mask{PLCOperandExpression=xxx_PLC_VAR_AtFloor1, PLCOperandTag=AtFloor1, PLCBlockType=XIO, PLCPOUType=Contact}
      mask prompts: PLCOperandTag "Operand Tag:"
      mask init:
      | slplc.callbacks.initInstruction(gcb);
      settings: AttributesFormatString=%<PLCOperandTag>
      mask Help: web([docroot '/plccoder/ref/xio' '.html']);
      mask DialogControl PLCBlockTitle Prompt: Examine If Open (XIO)
  XIO24 : Subsystem  Priority=9  TreatAsAtomicUnit=on  mask{PLCOperandExpression=xxx_PLC_VAR_AtFloor2, PLCOperandTag=AtFloor2, PLCBlockType=XIO, PLCPOUType=Contact}
      mask prompts: PLCOperandTag "Operand Tag:"
      mask init:
      | slplc.callbacks.initInstruction(gcb);
      settings: AttributesFormatString=%<PLCOperandTag>
      mask Help: web([docroot '/plccoder/ref/xio' '.html']);
      mask DialogControl PLCBlockTitle Prompt: Examine If Open (XIO)
  XIO25 : Subsystem  Priority=191  TreatAsAtomicUnit=on  mask{PLCOperandExpression=xxx_PLC_VAR_LSTDIRUP, PLCOperandTag=LSTDIRUP, PLCBlockType=XIO, PLCPOUType=Contact}
      mask prompts: PLCOperandTag "Operand Tag:"
      mask init:
      | slplc.callbacks.initInstruction(gcb);
      settings: AttributesFormatString=%<PLCOperandTag>
      mask Help: web([docroot '/plccoder/ref/xio' '.html']);
      mask DialogControl PLCBlockTitle Prompt: Examine If Open (XIO)
  XIO26 : Subsystem  Priority=192  TreatAsAtomicUnit=on  mask{PLCOperandExpression=xxx_PLC_VAR_MemoryGoUp, PLCOperandTag=MemoryGoUp, PLCBlockType=XIO, PLCPOUType=Contact}
      mask prompts: PLCOperandTag "Operand Tag:"
      mask init:
      | slplc.callbacks.initInstruction(gcb);
      settings: AttributesFormatString=%<PLCOperandTag>
      mask Help: web([docroot '/plccoder/ref/xio' '.html']);
      mask DialogControl PLCBlockTitle Prompt: Examine If Open (XIO)
  XIO27 : Subsystem  Priority=200  TreatAsAtomicUnit=on  mask{PLCOperandExpression=xxx_PLC_VAR_GOINGDN, PLCOperandTag=GOINGDN, PLCBlockType=XIO, PLCPOUType=Contact}
      mask prompts: PLCOperandTag "Operand Tag:"
      mask init:
      | slplc.callbacks.initInstruction(gcb);
      settings: AttributesFormatString=%<PLCOperandTag>
      mask Help: web([docroot '/plccoder/ref/xio' '.html']);
      mask DialogControl PLCBlockTitle Prompt: Examine If Open (XIO)
  XIO28 : Subsystem  Priority=260  TreatAsAtomicUnit=on  mask{PLCOperandExpression=xxx_PLC_VAR_RMPDNKIL, PLCOperandTag=RMPDNKIL, PLCBlockType=XIO, PLCPOUType=Contact}
      mask prompts: PLCOperandTag "Operand Tag:"
      mask init:
      | slplc.callbacks.initInstruction(gcb);
      settings: AttributesFormatString=%<PLCOperandTag>
      mask Help: web([docroot '/plccoder/ref/xio' '.html']);
      mask DialogControl PLCBlockTitle Prompt: Examine If Open (XIO)
  XIO29 : Subsystem  Priority=58  TreatAsAtomicUnit=on  mask{PLCOperandExpression=xxx_PLC_VAR_AtFloor2, PLCOperandTag=AtFloor2, PLCBlockType=XIO, PLCPOUType=Contact}
      mask prompts: PLCOperandTag "Operand Tag:"
      mask init:
      | slplc.callbacks.initInstruction(gcb);
      settings: AttributesFormatString=%<PLCOperandTag>
      mask Help: web([docroot '/plccoder/ref/xio' '.html']);
      mask DialogControl PLCBlockTitle Prompt: Examine If Open (XIO)
  XIO3 : Subsystem  Priority=130  TreatAsAtomicUnit=on  mask{PLCOperandExpression=xxx_PLC_VAR_AtFloor3, PLCOperandTag=AtFloor3, PLCBlockType=XIO, PLCPOUType=Contact}
      mask prompts: PLCOperandTag "Operand Tag:"
      mask init:
      | slplc.callbacks.initInstruction(gcb);
      settings: AttributesFormatString=%<PLCOperandTag>
      mask Help: web([docroot '/plccoder/ref/xio' '.html']);
      mask DialogControl PLCBlockTitle Prompt: Examine If Open (XIO)
  XIO30 : Subsystem  Priority=252  TreatAsAtomicUnit=on  mask{PLCOperandExpression=xxx_PLC_VAR_RMPUPKIL, PLCOperandTag=RMPUPKIL, PLCBlockType=XIO, PLCPOUType=Contact}
      mask prompts: PLCOperandTag "Operand Tag:"
      mask init:
      | slplc.callbacks.initInstruction(gcb);
      settings: AttributesFormatString=%<PLCOperandTag>
      mask Help: web([docroot '/plccoder/ref/xio' '.html']);
      mask DialogControl PLCBlockTitle Prompt: Examine If Open (XIO)
  XIO31 : Subsystem  Priority=30  TreatAsAtomicUnit=on  mask{PLCOperandExpression=xxx_PLC_VAR_AtFloor3, PLCOperandTag=AtFloor3, PLCBlockType=XIO, PLCPOUType=Contact}
      mask prompts: PLCOperandTag "Operand Tag:"
      mask init:
      | slplc.callbacks.initInstruction(gcb);
      settings: AttributesFormatString=%<PLCOperandTag>
      mask Help: web([docroot '/plccoder/ref/xio' '.html']);
      mask DialogControl PLCBlockTitle Prompt: Examine If Open (XIO)
  XIO32 : Subsystem  Priority=293  TreatAsAtomicUnit=on  mask{PLCOperandExpression=xxx_PLC_VAR_SENCHK, PLCOperandTag=SENCHK, PLCBlockType=XIO, PLCPOUType=Contact}
      mask prompts: PLCOperandTag "Operand Tag:"
      mask init:
      | slplc.callbacks.initInstruction(gcb);
      settings: AttributesFormatString=%<PLCOperandTag>
      mask Help: web([docroot '/plccoder/ref/xio' '.html']);
      mask DialogControl PLCBlockTitle Prompt: Examine If Open (XIO)
  XIO34 : Subsystem  Priority=90  TreatAsAtomicUnit=on  mask{PLCOperandExpression=xxx_PLC_VAR_AtFloor2, PLCOperandTag=AtFloor2, PLCBlockType=XIO, PLCPOUType=Contact}
      mask prompts: PLCOperandTag "Operand Tag:"
      mask init:
      | slplc.callbacks.initInstruction(gcb);
      settings: AttributesFormatString=%<PLCOperandTag>
      mask Help: web([docroot '/plccoder/ref/xio' '.html']);
      mask DialogControl PLCBlockTitle Prompt: Examine If Open (XIO)
  XIO4 : Subsystem  Priority=137  TreatAsAtomicUnit=on  mask{PLCOperandExpression=xxx_PLC_VAR_AtFloor1, PLCOperandTag=AtFloor1, PLCBlockType=XIO, PLCPOUType=Contact}
      mask prompts: PLCOperandTag "Operand Tag:"
      mask init:
      | slplc.callbacks.initInstruction(gcb);
      settings: AttributesFormatString=%<PLCOperandTag>
      mask Help: web([docroot '/plccoder/ref/xio' '.html']);
      mask DialogControl PLCBlockTitle Prompt: Examine If Open (XIO)
  XIO5 : Subsystem  Priority=146  TreatAsAtomicUnit=on  mask{PLCOperandExpression=xxx_PLC_VAR_AtFloor2, PLCOperandTag=AtFloor2, PLCBlockType=XIO, PLCPOUType=Contact}
      mask prompts: PLCOperandTag "Operand Tag:"
      mask init:
      | slplc.callbacks.initInstruction(gcb);
      settings: AttributesFormatString=%<PLCOperandTag>
      mask Help: web([docroot '/plccoder/ref/xio' '.html']);
      mask DialogControl PLCBlockTitle Prompt: Examine If Open (XIO)
  XIO6 : Subsystem  Priority=153  TreatAsAtomicUnit=on  mask{PLCOperandExpression=xxx_PLC_VAR_AtFloor3, PLCOperandTag=AtFloor3, PLCBlockType=XIO, PLCPOUType=Contact}
      mask prompts: PLCOperandTag "Operand Tag:"
      mask init:
      | slplc.callbacks.initInstruction(gcb);
      settings: AttributesFormatString=%<PLCOperandTag>
      mask Help: web([docroot '/plccoder/ref/xio' '.html']);
      mask DialogControl PLCBlockTitle Prompt: Examine If Open (XIO)
  XIO7 : Subsystem  Priority=160  TreatAsAtomicUnit=on  mask{PLCOperandExpression=xxx_PLC_VAR_AtFloor2, PLCOperandTag=AtFloor2, PLCBlockType=XIO, PLCPOUType=Contact}
      mask prompts: PLCOperandTag "Operand Tag:"
      mask init:
      | slplc.callbacks.initInstruction(gcb);
      settings: AttributesFormatString=%<PLCOperandTag>
      mask Help: web([docroot '/plccoder/ref/xio' '.html']);
      mask DialogControl PLCBlockTitle Prompt: Examine If Open (XIO)
  XIO8 : Subsystem  Priority=161  TreatAsAtomicUnit=on  mask{PLCOperandExpression=xxx_PLC_VAR_AtFloor3, PLCOperandTag=AtFloor3, PLCBlockType=XIO, PLCPOUType=Contact}
      mask prompts: PLCOperandTag "Operand Tag:"
      mask init:
      | slplc.callbacks.initInstruction(gcb);
      settings: AttributesFormatString=%<PLCOperandTag>
      mask Help: web([docroot '/plccoder/ref/xio' '.html']);
      mask DialogControl PLCBlockTitle Prompt: Examine If Open (XIO)
  XIO9 : Subsystem  Priority=165  TreatAsAtomicUnit=on  mask{PLCOperandExpression=xxx_PLC_VAR_AtFloor3, PLCOperandTag=AtFloor3, PLCBlockType=XIO, PLCPOUType=Contact}
      mask prompts: PLCOperandTag "Operand Tag:"
      mask init:
      | slplc.callbacks.initInstruction(gcb);
      settings: AttributesFormatString=%<PLCOperandTag>
      mask Help: web([docroot '/plccoder/ref/xio' '.html']);
      mask DialogControl PLCBlockTitle Prompt: Examine If Open (XIO)
  wires:
  XIC16/1(RungOut) -> Junction4/2(RungIn2)
  XIC11/1(RungOut) -> Junction3/1(RungIn1)
  Junction6/1(RungOut) -> Junction5/2(RungIn2)
  Junction5/1(RungOut) -> XIO5/1(RungIn)
  OTE10/1(RungOut) -> Rung Terminal11/1(RungIn)
  XIO12/1(RungOut) -> Junction11/2(RungIn2)
  XIC26/1(RungOut) -> XIC28/1(RungIn), XIC29/1(RungIn), XIC30/1(RungIn), XIC27/1(RungIn)
  Junction11/1(RungOut) -> OTE10/1(RungIn)
  XIC15/1(RungOut) -> Junction4/1(RungIn1)
  XIC3/1(RungOut) -> Junction1/1(RungIn1)
  OTE9/1(RungOut) -> Rung Terminal10/1(RungIn)
  XIO4/1(RungOut) -> OTE4/1(RungIn)
  OTE2/1(RungOut) -> Rung Terminal2/1(RungIn)
  XIO2/1(RungOut) -> OTE2/1(RungIn)
  XIC22/1(RungOut) -> Junction8/1(RungIn1)
  OTE/1(RungOut) -> Rung Terminal1/1(RungIn)
  XIO/1(RungOut) -> OTE/1(RungIn)
  OTE6/1(RungOut) -> Rung Terminal6/1(RungIn)
  Junction8/1(RungOut) -> XIO7/1(RungIn)
  XIO6/1(RungOut) -> OTE6/1(RungIn)
  XIC23/1(RungOut) -> Junction8/2(RungIn2)
  XIO5/1(RungOut) -> OTE5/1(RungIn)
  XIC14/1(RungOut) -> XIC16/1(RungIn), XIC15/1(RungIn)
  OTE5/1(RungOut) -> Rung Terminal5/1(RungIn)
  Junction12/1(RungOut) -> XIO10/1(RungIn)
  XIC2/1(RungOut) -> XIC4/1(RungIn), XIC3/1(RungIn)
  Junction20/1(RungOut) -> XIO/1(RungIn)
  XIC10/1(RungOut) -> XIC12/1(RungIn), XIC11/1(RungIn)
  OTE3/1(RungOut) -> Rung Terminal3/1(RungIn)
  XIC30/1(RungOut) -> Junction13/2(RungIn2)
  XIC29/1(RungOut) -> Junction13/1(RungIn1)
  Junction3/1(RungOut) -> XIO3/1(RungIn)
  XIC27/1(RungOut) -> Junction12/1(RungIn1)
  XIO11/1(RungOut) -> Junction11/1(RungIn1)
  Junction7/1(RungOut) -> XIO6/1(RungIn)
  XIC9/1(RungOut) -> Junction5/1(RungIn1)
  XIC13/1(RungOut) -> Junction6/1(RungIn1)
  XIC17/1(RungOut) -> Junction6/2(RungIn2)
  XIC5/1(RungOut) -> XIC9/1(RungIn), XIC17/1(RungIn), XIC13/1(RungIn)
  OTE1/1(RungOut) -> Rung Terminal/1(RungIn)
  Junction2/1(RungOut) -> XIO2/1(RungIn)
  XIO3/1(RungOut) -> OTE3/1(RungIn)
  Junction9/1(RungOut) -> OTE9/1(RungIn)
  XIC21/1(RungOut) -> XIC22/1(RungIn), XIC25/1(RungIn), XIC24/1(RungIn), XIC23/1(RungIn)
  XIO8/1(RungOut) -> Junction9/1(RungIn1)
  Junction10/1(RungOut) -> XIO9/1(RungIn)
  XIC25/1(RungOut) -> Junction10/2(RungIn2)
  XIO10/1(RungOut) -> XIO11/1(RungIn)
  Junction13/1(RungOut) -> XIO12/1(RungIn)
  XIC28/1(RungOut) -> Junction12/2(RungIn2)
  XIO7/1(RungOut) -> XIO8/1(RungIn)
  OTE4/1(RungOut) -> Rung Terminal4/1(RungIn)
  XIC19/1(RungOut) -> Junction7/1(RungIn1)
  XIC7/1(RungOut) -> Junction2/1(RungIn1)
  XIC20/1(RungOut) -> Junction7/2(RungIn2)
  XIC18/1(RungOut) -> XIC19/1(RungIn), XIC20/1(RungIn)
  XIC8/1(RungOut) -> Junction2/2(RungIn2)
  XIO1/1(RungOut) -> OTE1/1(RungIn)
  XIC6/1(RungOut) -> XIC7/1(RungIn), XIC8/1(RungIn)
  XIC1/1(RungOut) -> Junction20/2(RungIn2)
  Junction1/1(RungOut) -> XIO1/1(RungIn)
  XIC4/1(RungOut) -> Junction1/2(RungIn2)
  XIC24/1(RungOut) -> Junction10/1(RungIn1)
  Junction4/1(RungOut) -> XIO4/1(RungIn)
  XIO9/1(RungOut) -> Junction9/2(RungIn2)
  XIC12/1(RungOut) -> Junction3/2(RungIn2)
  MOV3/1(RungOut) -> Rung Terminal17/1(RungIn)
  Variable Read3/1(VarOut) -> MOV3/2(src)
  MOV1/1(RungOut) -> Rung Terminal15/1(RungIn)
  MOV2/2(dest) -> Variable Write2/1(VarIn)
  Variable Read2/1(VarOut) -> MOV2/2(src)
  MOV1/2(dest) -> Variable Write1/1(VarIn)
  MOV2/1(RungOut) -> Rung Terminal16/1(RungIn)
  Variable Read1/1(VarOut) -> MOV1/2(src)
  XIO15/1(RungOut) -> MOV1/1(RungIn)
  MOV3/2(dest) -> Variable Write3/1(VarIn)
  XIC62/1(RungOut) -> Junction23/1(RungIn1)
  Junction23/1(RungOut) -> OTE18/1(RungIn)
  Junction22/1(RungOut) -> OTE17/1(RungIn)
  XIC60/1(RungOut) -> Junction22/1(RungIn1)
  Junction24/1(RungOut) -> MOV2/1(RungIn)
  XIC66/1(RungOut) -> Junction25/1(RungIn1)
  XIC64/1(RungOut) -> Junction26/1(RungIn1)
  XIO16/1(RungOut) -> MOV3/1(RungIn)
  Variable Read4/1(VarOut) -> EQU/2(srcA)
  Variable Read5/1(VarOut) -> EQU/3(srcB)
  XIC74/1(RungOut) -> XIO19/1(RungIn)
  EQU/1(RungOut) -> OTE23/1(RungIn)
  OTE23/1(RungOut) -> Rung Terminal18/1(RungIn)
  OTE24/1(RungOut) -> Rung Terminal19/1(RungIn)
  EQU1/1(RungOut) -> OTE24/1(RungIn)
  XIC75/1(RungOut) -> XIO20/1(RungIn)
  Variable Read7/1(VarOut) -> EQU1/3(srcB)
  Variable Read6/1(VarOut) -> EQU1/2(srcA)
  Variable Read8/1(VarOut) -> EQU2/2(srcA)
  Variable Read9/1(VarOut) -> EQU2/3(srcB)
  XIC76/1(RungOut) -> XIO22/1(RungIn)
  EQU2/1(RungOut) -> OTE25/1(RungIn)
  OTE25/1(RungOut) -> Rung Terminal20/1(RungIn)
  XIC87/1(RungOut) -> XIO13/1(RungIn)
  OTE19/1(RungOut) -> Rung Terminal21/1(RungIn)
  OTE20/1(RungOut) -> Rung Terminal22/1(RungIn)
  XIC79/1(RungOut) -> XIO15/1(RungIn)
  XIC81/1(RungOut) -> XIC82/1(RungIn)
  XIC84/1(RungOut) -> XIO14/1(RungIn)
  Junction25/1(RungOut) -> OTE20/1(RungIn)
  XIC69/1(RungOut) -> XIC86/1(RungIn)
  Junction26/1(RungOut) -> OTE19/1(RungIn)
  OTE17/1(RungOut) -> Rung Terminal23/1(RungIn)
  OTE18/1(RungOut) -> Rung Terminal24/1(RungIn)
  XIC77/1(RungOut) -> XIC67/1(RungIn), XIC66/1(RungIn)
  XIC43/1(RungOut) -> XIO16/1(RungIn)
  XIC82/1(RungOut) -> XIC63/1(RungIn), XIC62/1(RungIn)
  XIC70/1(RungOut) -> XIC61/1(RungIn), XIC60/1(RungIn)
  XIC45/1(RungOut) -> XIC43/1(RungIn)
  XIC78/1(RungOut) -> XIC77/1(RungIn)
  XIC80/1(RungOut) -> XIC79/1(RungIn)
  XIO13/1(RungOut) -> Junction24/1(RungIn1)
  XIO14/1(RungOut) -> Junction24/2(RungIn2)
  XIC83/1(RungOut) -> XIC84/1(RungIn), XIC87/1(RungIn)
  XIO18/1(RungOut) -> EQU/1(RungIn)
  XIO19/1(RungOut) -> XIO18/1(RungIn)
  XIO20/1(RungOut) -> XIO21/1(RungIn)
  XIO21/1(RungOut) -> EQU1/1(RungIn)
  XIO22/1(RungOut) -> XIO34/1(RungIn)
  XIO34/1(RungOut) -> EQU2/1(RungIn)
  XIC67/1(RungOut) -> Junction25/2(RungIn2)
  XIC65/1(RungOut) -> Junction26/2(RungIn2)
  XIO23/1(RungOut) -> XIC65/1(RungIn), XIC64/1(RungIn)
  XIC63/1(RungOut) -> Junction23/2(RungIn2)
  XIC61/1(RungOut) -> Junction22/2(RungIn2)
  XIC88/1(RungOut) -> Junction27/2(RungIn2)
  Junction27/1(RungOut) -> OTE15/1(RungIn)
  OTE15/1(RungOut) -> Rung Terminal25/1(RungIn)
  XIC85/1(RungOut) -> Junction27/1(RungIn1)
  XIC91/1(RungOut) -> Junction28/2(RungIn2)
  Junction28/1(RungOut) -> OTE16/1(RungIn)
  OTE16/1(RungOut) -> Rung Terminal26/1(RungIn)
  XIC90/1(RungOut) -> Junction28/1(RungIn1)
  XIC94/1(RungOut) -> Junction32/2(RungIn2)
  OTE21/1(RungOut) -> Rung Terminal27/1(RungIn)
  Junction32/1(RungOut) -> OTE21/1(RungIn)
  XIC93/1(RungOut) -> Junction32/1(RungIn1)
  XIC96/1(RungOut) -> Junction33/2(RungIn2)
  OTE22/1(RungOut) -> Rung Terminal28/1(RungIn)
  XIC95/1(RungOut) -> Junction33/1(RungIn1)
  Junction33/1(RungOut) -> OTE22/1(RungIn)
  XIC71/1(RungOut) -> XIO29/1(RungIn)
  XIO29/1(RungOut) -> XIC88/1(RungIn), XIC85/1(RungIn)
  XIC86/1(RungOut) -> XIC91/1(RungIn), XIC90/1(RungIn)
  XIC68/1(RungOut) -> XIO23/1(RungIn)
  XIC72/1(RungOut) -> XIO31/1(RungIn)
  XIO31/1(RungOut) -> XIC94/1(RungIn), XIC93/1(RungIn)
  XIC59/1(RungOut) -> XIC70/1(RungIn)
  XIC58/1(RungOut) -> XIO24/1(RungIn)
  XIO24/1(RungOut) -> XIC96/1(RungIn), XIC95/1(RungIn)
  XIC73/1(RungOut) -> XIC44/1(RungIn)
  XIC44/1(RungOut) -> XIO17/1(RungIn), XIC89/1(RungIn)
  XIC89/1(RungOut) -> Junction/1(RungIn1)
  XIO17/1(RungOut) -> Junction/2(RungIn2)
  Junction/1(RungOut) -> OTE26/1(RungIn)
  OTE26/1(RungOut) -> Rung Terminal29/1(RungIn)
  Junction18/1(RungOut) -> OTE27/1(RungIn)
  XIC98/1(RungOut) -> XIC97/1(RungIn)
  XIO25/1(RungOut) -> Junction18/1(RungIn1)
  XIC97/1(RungOut) -> XIO26/1(RungIn), XIO25/1(RungIn)
  XIO26/1(RungOut) -> Junction18/2(RungIn2)
  OTE27/1(RungOut) -> Rung Terminal30/1(RungIn)
  XIC99/1(RungOut) -> XIC100/1(RungIn), XIC92/1(RungIn)
  XIC100/1(RungOut) -> Junction29/2(RungIn2)
  XIC92/1(RungOut) -> Junction29/1(RungIn1)
  Junction29/1(RungOut) -> OTE28/1(RungIn)
  OTE28/1(RungOut) -> Rung Terminal31/1(RungIn)
  OTE7/1(RungOut) -> Rung Terminal8/1(RungIn)
  Junction16/1(RungOut) -> Junction30/1(RungIn1)
  Junction21/1(RungOut) -> XIC49/1(RungIn)
  XIC51/1(RungOut) -> Junction14/1(RungIn1)
  Junction14/1(RungOut) -> XIC46/1(RungIn)
  XIC48/1(RungOut) -> Junction15/2(RungIn2)
  Junction30/1(RungOut) -> OTE7/1(RungIn)
  XIC46/1(RungOut) -> Junction17/2(RungIn2)
  XIC52/1(RungOut) -> Junction19/2(RungIn2)
  Junction19/1(RungOut) -> XIC47/1(RungIn)
  XIC57/1(RungOut) -> Junction14/2(RungIn2)
  XIC35/1(RungOut) -> Junction15/1(RungIn1)
  XIC37/1(RungOut) -> Junction19/1(RungIn1)
  XIC55/1(RungOut) -> XIC57/1(RungIn), XIC51/1(RungIn), XIC48/1(RungIn), XIC35/1(RungIn)
  XIC47/1(RungOut) -> Junction16/1(RungIn1)
  XIC56/1(RungOut) -> XIC55/1(RungIn), XIC53/1(RungIn)
  XIC50/1(RungOut) -> Junction17/1(RungIn1)
  XIC54/1(RungOut) -> Junction21/1(RungIn1)
  XIC36/1(RungOut) -> Junction21/2(RungIn2)
  XIC53/1(RungOut) -> XIC37/1(RungIn), XIC52/1(RungIn), XIC36/1(RungIn), XIC54/1(RungIn)
  Junction15/1(RungOut) -> XIC50/1(RungIn)
  Junction17/1(RungOut) -> Junction30/2(RungIn2)
  XIC49/1(RungOut) -> Junction16/2(RungIn2)
  Junction31/1(RungOut) -> XIO27/1(RungIn)
  XIC33/1(RungOut) -> Junction31/1(RungIn1)
  XIC32/1(RungOut) -> Junction31/2(RungIn2)
  XIC31/1(RungOut) -> XIC33/1(RungIn), XIC32/1(RungIn)
  XIO27/1(RungOut) -> OTE8/1(RungIn)
  OTE8/1(RungOut) -> Rung Terminal7/1(RungIn)
  TON/1(EN) -> OTE11/1(RungIn)
  OTE11/1(RungOut) -> Rung Terminal9/1(RungIn)
  XIC38/1(RungOut) -> XIC40/1(RungIn), XIC39/1(RungIn)
  XIC40/1(RungOut) -> Junction34/2(RungIn2)
  XIC39/1(RungOut) -> Junction34/1(RungIn1)
  Junction34/1(RungOut) -> XIO30/1(RungIn)
  XIO30/1(RungOut) -> OTE12/1(RungIn)
  OTE12/1(RungOut) -> Rung Terminal12/1(RungIn)
  XIC/1(RungOut) -> Junction20/1(RungIn1)
  XIC34/1(RungOut) -> EQU3/1(RungIn)
  EQU3/1(RungOut) -> TON/1(RungIn)
  XIC42/1(RungOut) -> XIC34/1(RungIn)
  Variable Read/1(VarOut) -> EQU3/2(srcA)
  Constant/1 -> EQU3/3(srcB)
  XIC102/1(RungOut) -> XIC38/1(RungIn)
  XIC105/1(RungOut) -> XIC107/1(RungIn)
  Constant2/1 -> SUB/3(srcB)
  SUB/1(RungOut) -> Rung Terminal32/1(RungIn)
  SUB/2(dest) -> Variable Write5/1(VarIn)
  Variable Read11/1(VarOut) -> SUB/2(srcA)
  XIC110/1(RungOut) -> SUB/1(RungIn)
  OTE13/1(RungOut) -> Rung Terminal14/1(RungIn)
  XIO28/1(RungOut) -> OTE13/1(RungIn)
  Junction35/1(RungOut) -> XIO28/1(RungIn)
  XIC108/1(RungOut) -> Junction35/1(RungIn1)
  XIC109/1(RungOut) -> Junction35/2(RungIn2)
  XIC107/1(RungOut) -> XIC108/1(RungIn), XIC109/1(RungIn)
  OTE14/1(RungOut) -> Rung Terminal13/1(RungIn)
  XIC101/1(RungOut) -> XIC41/1(RungIn)
  XIC41/1(RungOut) -> OTE29/1(RungIn), OTE14/1(RungIn)
  OTE29/1(RungOut) -> Rung Terminal33/1(RungIn)
  Constant1/1 -> ADD/3(srcB)
  Variable Read10/1(VarOut) -> ADD/2(srcA)
  ADD/1(RungOut) -> Rung Terminal34/1(RungIn)
  ADD/2(dest) -> Variable Write4/1(VarIn)
  Power Rail Start/1(PowerOut) -> XIC117/1(RungIn), XIC118/1(RungIn), Power Rail Terminal/1(PowerIn), XIC103/1(RungIn), XIC115/1(RungIn), XIC113/1(RungIn), XIC98/1(RungIn), XIC99/1(RungIn), XIC56/1(RungIn), XIC101/1(RungIn), XIC102/1(RungIn), XIC111/1(RungIn), XIC106/1(RungIn), XIC105/1(RungIn), XIC42/1(RungIn), XIC31/1(RungIn), XIC73/1(RungIn), XIC26/1(RungIn), XIC21/1(RungIn), XIC18/1(RungIn), XIC5/1(RungIn), XIC14/1(RungIn), XIC10/1(RungIn), XIC6/1(RungIn), XIC2/1(RungIn), XIC74/1(RungIn), XIC75/1(RungIn), XIC76/1(RungIn), XIC80/1(RungIn), XIC83/1(RungIn), XIC45/1(RungIn), XIC71/1(RungIn), XIC78/1(RungIn), XIC69/1(RungIn), XIC68/1(RungIn), XIC72/1(RungIn), XIC81/1(RungIn), XIC59/1(RungIn), XIC58/1(RungIn), XIC1/1(RungIn), XIC/1(RungIn)
  XIC111/1(RungOut) -> XIC112/1(RungIn)
  XIC106/1(RungOut) -> XIC110/1(RungIn)
  XIC103/1(RungOut) -> XIC104/1(RungIn)
  XIC104/1(RungOut) -> XIO32/1(RungIn)
  XIO32/1(RungOut) -> MUL/1(RungIn)
  MUL/1(RungOut) -> Rung Terminal35/1(RungIn)
  Constant3/1 -> MUL/3(srcB)
  Variable Read12/1(VarOut) -> MUL/2(srcA)
  MUL/2(dest) -> Variable Write6/1(VarIn)
  XIC112/1(RungOut) -> LEQ/1(RungIn)
  Variable Read13/1(VarOut) -> LEQ/2(srcA)
  Constant4/1 -> LEQ/3(srcB)
  LEQ/1(RungOut) -> OTE30/1(RungIn)
  OTE30/1(RungOut) -> Rung Terminal36/1(RungIn)
  XIC113/1(RungOut) -> XIC114/1(RungIn)
  XIC114/1(RungOut) -> ADD/1(RungIn)
  OTE31/1(RungOut) -> Rung Terminal37/1(RungIn)
  Constant5/1 -> GRT/3(srcB)
  Variable Read14/1(VarOut) -> GRT/2(srcA)
  XIC116/1(RungOut) -> GRT/1(RungIn)
  XIC115/1(RungOut) -> XIC116/1(RungIn)
  GRT/1(RungOut) -> OTE31/1(RungIn)
  MOV/1(RungOut) -> Rung Terminal38/1(RungIn)
  XIC117/1(RungOut) -> MOV/1(RungIn)
  Variable Read15/1(VarOut) -> MOV/2(src)
  MOV/2(dest) -> Variable Write7/1(VarIn)
  MOV4/2(dest) -> Variable Write8/1(VarIn)
  XIC118/1(RungOut) -> MOV4/1(RungIn)
  MOV4/1(RungOut) -> Rung Terminal39/1(RungIn)
  Variable Read16/1(VarOut) -> MOV4/2(src)
